simulink model "LinearSolver_System"  (R2021a)
settings: Solver=VariableStepAuto  StartTime=0.0  StopTime=1000  RelTol=1e-3
undefined symbols (not defined in the file or in its folder): AXI4, Lite
libraries: hdlBasic x415, xbsIndex_r4 x1
(part 4 of 4)

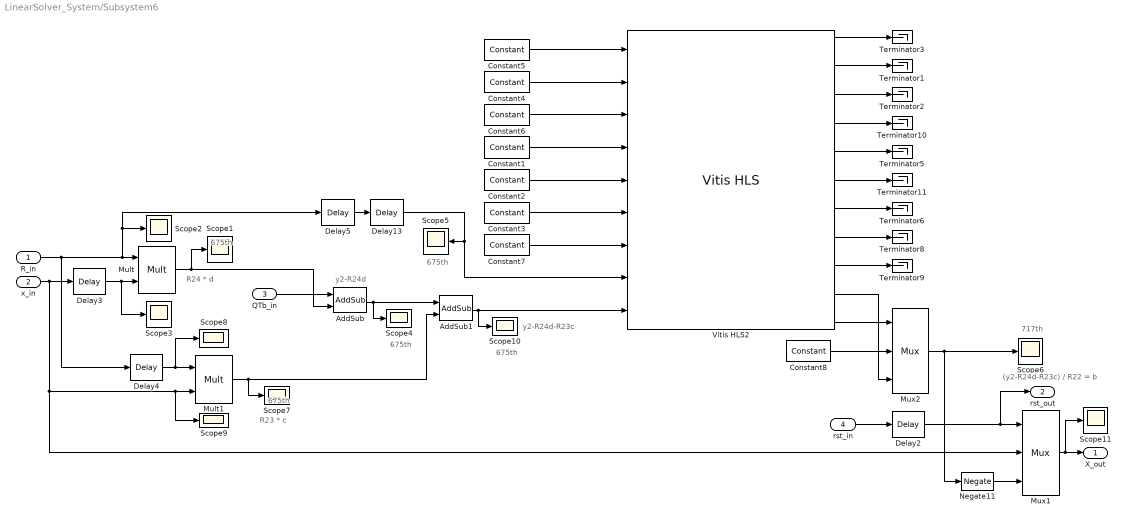
== system LinearSolver_System/Subsystem6 ==
  note: 717th
  note: R24 * d
  note: y2-R24d-R23c
  note: 675th
  note: 675th
  note: (y2-R24d-R23c) / R22 = b
  note: R23 * c
  note: 675th
  note: 675th
  note: 675th
  note: y2-R24d
  R_in : Inport
  x_in : Inport  Port=2
  QTb_in : Inport  Port=3
  rst_in : Inport  Port=4
  AddSub : hdlBasic/AddSub  mode=Subtraction  use_carryin=off  use_carryout=off  en=off  latency=0  precision=User Defined  arith_type="Signed  (2's comp)"  n_bits=16  bin_pt=13  quantization="Round  (unbiased: +/- Inf)"  overflow=Saturate  use_behavioral_HDL=off  hw_selection=Fabric  pipelined=off  XmcBlockStatus=1  maskContainerNames=tabcontainer1  block_type=addsub  block_config=sysgen:Addsub_config
  AddSub1 : hdlBasic/AddSub  mode=Subtraction  use_carryin=off  use_carryout=off  en=off  latency=0  precision=User Defined  arith_type="Signed  (2's comp)"  n_bits=16  bin_pt=13  quantization="Round  (unbiased: +/- Inf)"  overflow=Saturate  use_behavioral_HDL=off  hw_selection=Fabric  pipelined=off  XmcBlockStatus=1  maskContainerNames=tabcontainer1  block_type=addsub  block_config=sysgen:Addsub_config
  Constant{1..3,8} (4 alike) : hdlBasic/Constant  const=0.0  gui_display_data_type=Fixed-point  arith_type=Signed (2's comp)  n_bits=16  bin_pt=13  preci_type=Single  exp_width=8  frac_width=24  explicit_period=off  period=1  XmcBlockStatus=1  maskContainerNames=tabcontainer1  block_type=constant  block_config=sysgen:Constant_config
  Constant4 : hdlBasic/Constant  const=1.0  gui_display_data_type=Boolean  arith_type=Boolean  n_bits=16  bin_pt=14  preci_type=Single  exp_width=8  frac_width=24  explicit_period=off  period=1  XmcBlockStatus=1  maskContainerNames=tabcontainer1  block_type=constant  block_config=sysgen:Constant_config
  Constant5 : hdlBasic/Constant  const=0  gui_display_data_type=Boolean  arith_type=Boolean  n_bits=16  bin_pt=14  preci_type=Single  exp_width=8  frac_width=24  explicit_period=off  period=1  XmcBlockStatus=1  maskContainerNames=tabcontainer1  block_type=constant  block_config=sysgen:Constant_config
  Constant6 : hdlBasic/Constant  const=0  gui_display_data_type=Boolean  arith_type=Boolean  n_bits=16  bin_pt=13  preci_type=Single  exp_width=8  frac_width=24  explicit_period=off  period=1  XmcBlockStatus=1  maskContainerNames=tabcontainer1  block_type=constant  block_config=sysgen:Constant_config
  Constant7 : hdlBasic/Constant  const=0.0  gui_display_data_type=Fixed-point  arith_type=Signed (2's comp)  n_bits=16  bin_pt=0  preci_type=Single  exp_width=8  frac_width=24  explicit_period=off  period=1  XmcBlockStatus=1  maskContainerNames=tabcontainer1  block_type=constant  block_config=sysgen:Constant_config
  Delay{2..5,13} (5 alike) : hdlBasic/Delay  rst=off  en=off  latency=42  reg_retiming=off  XmcBlockStatus=1  maskContainerNames=group1  block_type=delay  block_config=sysgen:Delay_config
  Mult : hdlBasic/Mult  precision=User Defined  arith_type="Signed  (2's comp)"  n_bits=16  bin_pt=13  quantization="Round  (unbiased: +/- Inf)"  overflow=Saturate  en=off  latency=0  use_behavioral_HDL=off  opt=Speed  use_embedded=on  optimum_pipeline=off  pipeline=on  use_rpm=on  placement_style=Triangular  XmcBlockStatus=1  maskContainerNames=group1  block_type=mult  block_config=sysgen:Mult_config
  Mult1 : hdlBasic/Mult  precision=User Defined  arith_type="Signed  (2's comp)"  n_bits=16  bin_pt=13  quantization="Round  (unbiased: +/- Inf)"  overflow=Saturate  en=off  latency=0  use_behavioral_HDL=off  opt=Speed  use_embedded=on  optimum_pipeline=off  pipeline=on  use_rpm=on  placement_style=Triangular  XmcBlockStatus=1  maskContainerNames=group1  block_type=mult  block_config=sysgen:Mult_config
  Mux1 : hdlBasic/Mux  inputs=2  en=off  latency=0  precision=User Defined  arith_type="Signed  (2's comp)"  n_bits=16  bin_pt=13  quantization="Round  (unbiased: +/- Inf)"  overflow=Saturate  XmcBlockStatus=1  maskContainerNames=tabcontainer1  block_type=mux  block_config=sysgen:Mux_config
  Mux2 : hdlBasic/Mux  inputs=2  en=off  latency=0  precision=User Defined  arith_type="Signed  (2's comp)"  n_bits=16  bin_pt=13  quantization="Round  (unbiased: +/- Inf)"  overflow=Saturate  XmcBlockStatus=1  maskContainerNames=tabcontainer1  block_type=mux  block_config=sysgen:Mux_config
  Negate11 : hdlBasic/Negate  precision=User Defined  arith_type="Signed  (2's comp)"  n_bits=16  bin_pt=13  quantization=Truncate  overflow=Wrap  en=off  latency=0  XmcBlockStatus=1  maskContainerNames=tabcontainer1  block_type=negate  block_config=sysgen:Negate_config
  Scope{1..11} (11 alike) : Scope
  Terminator{1..3,5..6,8..11} (9 alike) : Terminator
  Vitis HLS2 : hdlBasic/Vitis HLS  anytable='..\Vitis_HLS\project6_final_hls_mc\solution2_add_back_substitution'  fast_sim=off  display_datatype=off  rate_propagation_method=Simulink system period  model_file_path=''  latency=1  block_type=vitis_hls
      settings: infoedit=This block allows including C,C++ and SystemC source files in System Generator for DSP designs.
  X_out : Outport
  rst_out : Outport  Port=2
  wires:
  Constant4/1 -> Vitis HLS2/2
  Vitis HLS2/4 -> Terminator10/1
  Constant2/1 -> Vitis HLS2/5
  Constant3/1 -> Vitis HLS2/6
  Constant5/1 -> Vitis HLS2/1
  Vitis HLS2/2 -> Terminator1/1
  Vitis HLS2/8 -> Terminator8/1
  Vitis HLS2/9 -> Terminator9/1
  Vitis HLS2/1 -> Terminator3/1
  Constant1/1 -> Vitis HLS2/4
  Constant6/1 -> Vitis HLS2/3
  Constant7/1 -> Vitis HLS2/7
  Vitis HLS2/3 -> Terminator2/1
  Vitis HLS2/5 -> Terminator5/1
  Vitis HLS2/7 -> Terminator6/1
  Vitis HLS2/6 -> Terminator11/1
  QTb_in/1 -> AddSub/1
  R_in/1 -> Delay4/1, Delay5/1, Scope2/1, Mult/1
  Mult/1 -> AddSub/2, Scope1/1
  AddSub/1 -> AddSub1/1, Scope4/1
  Delay13/1 -> Vitis HLS2/8, Scope5/1
  Constant8/1 -> Mux2/2
  Vitis HLS2/10 -> Mux2/3
  Vitis HLS2/11 -> Mux2/1
  rst_in/1 -> Delay2/1
  Delay2/1 -> rst_out/1, Mux1/1
  x_in/1 -> Mux1/2, Scope9/1, Mult1/2, Delay3/1
  Delay3/1 -> Scope3/1, Mult/2
  Mult1/1 -> AddSub1/2, Scope7/1
  Delay4/1 -> Scope8/1, Mult1/1
  AddSub1/1 -> Scope10/1, Vitis HLS2/9
  Delay5/1 -> Delay13/1
  Mux1/1 -> Scope11/1, X_out/1
  Mux2/1 -> Negate11/1, Scope6/1
  Negate11/1 -> Mux1/3

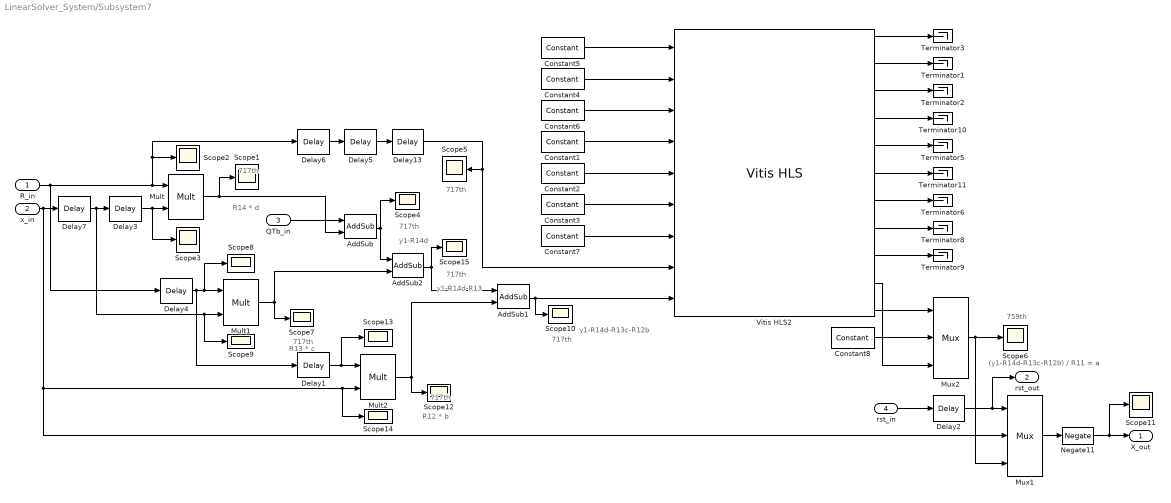
== system LinearSolver_System/Subsystem7 ==
  note: 759th
  note: R14 * d
  note: y1-R14d-R13c-R12b
  note: 717th
  note: 717th
  note: (y1-R14d-R13c-R12b) / R11 = a
  note: R13 * c
  note: 717th
  note: 717th
  note: 717th
  note: y1-R14d
  note: R12 * b
  note: 717th
  note: 717th
  note: y1-R14d-R13
  R_in : Inport
  x_in : Inport  Port=2
  QTb_in : Inport  Port=3
  rst_in : Inport  Port=4
  AddSub : hdlBasic/AddSub  mode=Subtraction  use_carryin=off  use_carryout=off  en=off  latency=0  precision=User Defined  arith_type="Signed  (2's comp)"  n_bits=16  bin_pt=13  quantization="Round  (unbiased: +/- Inf)"  overflow=Saturate  use_behavioral_HDL=off  hw_selection=Fabric  pipelined=off  XmcBlockStatus=1  maskContainerNames=tabcontainer1  block_type=addsub  block_config=sysgen:Addsub_config
  AddSub1 : hdlBasic/AddSub  mode=Subtraction  use_carryin=off  use_carryout=off  en=off  latency=0  precision=User Defined  arith_type="Signed  (2's comp)"  n_bits=16  bin_pt=13  quantization="Round  (unbiased: +/- Inf)"  overflow=Saturate  use_behavioral_HDL=off  hw_selection=Fabric  pipelined=off  XmcBlockStatus=1  maskContainerNames=tabcontainer1  block_type=addsub  block_config=sysgen:Addsub_config
  AddSub2 : hdlBasic/AddSub  mode=Subtraction  use_carryin=off  use_carryout=off  en=off  latency=0  precision=User Defined  arith_type="Signed  (2's comp)"  n_bits=16  bin_pt=13  quantization="Round  (unbiased: +/- Inf)"  overflow=Saturate  use_behavioral_HDL=off  hw_selection=Fabric  pipelined=off  XmcBlockStatus=1  maskContainerNames=tabcontainer1  block_type=addsub  block_config=sysgen:Addsub_config
  Constant{1..3,8} (4 alike) : hdlBasic/Constant  const=0.0  gui_display_data_type=Fixed-point  arith_type=Signed (2's comp)  n_bits=16  bin_pt=13  preci_type=Single  exp_width=8  frac_width=24  explicit_period=off  period=1  XmcBlockStatus=1  maskContainerNames=tabcontainer1  block_type=constant  block_config=sysgen:Constant_config
  Constant4 : hdlBasic/Constant  const=1.0  gui_display_data_type=Boolean  arith_type=Boolean  n_bits=16  bin_pt=14  preci_type=Single  exp_width=8  frac_width=24  explicit_period=off  period=1  XmcBlockStatus=1  maskContainerNames=tabcontainer1  block_type=constant  block_config=sysgen:Constant_config
  Constant5 : hdlBasic/Constant  const=0  gui_display_data_type=Boolean  arith_type=Boolean  n_bits=16  bin_pt=14  preci_type=Single  exp_width=8  frac_width=24  explicit_period=off  period=1  XmcBlockStatus=1  maskContainerNames=tabcontainer1  block_type=constant  block_config=sysgen:Constant_config
  Constant6 : hdlBasic/Constant  const=0  gui_display_data_type=Boolean  arith_type=Boolean  n_bits=16  bin_pt=13  preci_type=Single  exp_width=8  frac_width=24  explicit_period=off  period=1  XmcBlockStatus=1  maskContainerNames=tabcontainer1  block_type=constant  block_config=sysgen:Constant_config
  Constant7 : hdlBasic/Constant  const=0.0  gui_display_data_type=Fixed-point  arith_type=Signed (2's comp)  n_bits=16  bin_pt=0  preci_type=Single  exp_width=8  frac_width=24  explicit_period=off  period=1  XmcBlockStatus=1  maskContainerNames=tabcontainer1  block_type=constant  block_config=sysgen:Constant_config
  Delay{1..7,13} (8 alike) : hdlBasic/Delay  rst=off  en=off  latency=42  reg_retiming=off  XmcBlockStatus=1  maskContainerNames=group1  block_type=delay  block_config=sysgen:Delay_config
  Mult : hdlBasic/Mult  precision=User Defined  arith_type="Signed  (2's comp)"  n_bits=16  bin_pt=13  quantization="Round  (unbiased: +/- Inf)"  overflow=Saturate  en=off  latency=0  use_behavioral_HDL=off  opt=Speed  use_embedded=on  optimum_pipeline=off  pipeline=on  use_rpm=on  placement_style=Triangular  XmcBlockStatus=1  maskContainerNames=group1  block_type=mult  block_config=sysgen:Mult_config
  Mult1 : hdlBasic/Mult  precision=User Defined  arith_type="Signed  (2's comp)"  n_bits=16  bin_pt=13  quantization="Round  (unbiased: +/- Inf)"  overflow=Saturate  en=off  latency=0  use_behavioral_HDL=off  opt=Speed  use_embedded=on  optimum_pipeline=off  pipeline=on  use_rpm=on  placement_style=Triangular  XmcBlockStatus=1  maskContainerNames=group1  block_type=mult  block_config=sysgen:Mult_config
  Mult2 : hdlBasic/Mult  precision=User Defined  arith_type="Signed  (2's comp)"  n_bits=16  bin_pt=13  quantization="Round  (unbiased: +/- Inf)"  overflow=Saturate  en=off  latency=0  use_behavioral_HDL=off  opt=Speed  use_embedded=on  optimum_pipeline=off  pipeline=on  use_rpm=on  placement_style=Triangular  XmcBlockStatus=1  maskContainerNames=group1  block_type=mult  block_config=sysgen:Mult_config
  Mux1 : hdlBasic/Mux  inputs=2  en=off  latency=0  precision=Full  arith_type="Signed  (2's comp)"  n_bits=16  bin_pt=13  quantization="Round  (unbiased: +/- Inf)"  overflow=Saturate  XmcBlockStatus=1  maskContainerNames=tabcontainer1  block_type=mux  block_config=sysgen:Mux_config
  Mux2 : hdlBasic/Mux  inputs=2  en=off  latency=0  precision=User Defined  arith_type="Signed  (2's comp)"  n_bits=16  bin_pt=13  quantization="Round  (unbiased: +/- Inf)"  overflow=Saturate  XmcBlockStatus=1  maskContainerNames=tabcontainer1  block_type=mux  block_config=sysgen:Mux_config
  Negate11 : hdlBasic/Negate  precision=User Defined  arith_type="Signed  (2's comp)"  n_bits=16  bin_pt=13  quantization=Truncate  overflow=Wrap  en=off  latency=0  XmcBlockStatus=1  maskContainerNames=tabcontainer1  block_type=negate  block_config=sysgen:Negate_config
  Scope{1..15} (15 alike) : Scope
  Terminator{1..3,5..6,8..11} (9 alike) : Terminator
  Vitis HLS2 : hdlBasic/Vitis HLS  anytable='..\Vitis_HLS\project6_final_hls_mc\solution2_add_back_substitution'  fast_sim=off  display_datatype=off  rate_propagation_method=Simulink system period  model_file_path=''  latency=1  block_type=vitis_hls
      settings: infoedit=This block allows including C,C++ and SystemC source files in System Generator for DSP designs.
  X_out : Outport
  rst_out : Outport  Port=2
  wires:
  Constant4/1 -> Vitis HLS2/2
  Vitis HLS2/4 -> Terminator10/1
  Constant2/1 -> Vitis HLS2/5
  Constant3/1 -> Vitis HLS2/6
  Constant5/1 -> Vitis HLS2/1
  Vitis HLS2/2 -> Terminator1/1
  Vitis HLS2/8 -> Terminator8/1
  Vitis HLS2/9 -> Terminator9/1
  Vitis HLS2/1 -> Terminator3/1
  Constant1/1 -> Vitis HLS2/4
  Constant6/1 -> Vitis HLS2/3
  Constant7/1 -> Vitis HLS2/7
  Vitis HLS2/3 -> Terminator2/1
  Vitis HLS2/5 -> Terminator5/1
  Vitis HLS2/7 -> Terminator6/1
  Vitis HLS2/6 -> Terminator11/1
  QTb_in/1 -> AddSub/1
  R_in/1 -> Delay6/1, Scope2/1, Mult/1, Delay4/1
  Mult/1 -> AddSub/2, Scope1/1
  AddSub/1 -> AddSub2/1, Scope4/1
  Delay13/1 -> Vitis HLS2/8, Scope5/1
  Constant8/1 -> Mux2/2
  Vitis HLS2/10 -> Mux2/3
  Vitis HLS2/11 -> Mux2/1
  rst_in/1 -> Delay2/1
  Delay2/1 -> rst_out/1, Mux1/1
  x_in/1 -> Scope14/1, Mult2/2, Mux1/2, Delay7/1
  Delay3/1 -> Scope3/1, Mult/2
  Mult1/1 -> AddSub2/2, Scope7/1
  Delay4/1 -> Delay1/1, Scope8/1, Mult1/1
  AddSub1/1 -> Scope10/1, Vitis HLS2/9
  Delay5/1 -> Delay13/1
  Mult2/1 -> AddSub1/2, Scope12/1
  Delay1/1 -> Scope13/1, Mult2/1
  AddSub2/1 -> AddSub1/1, Scope15/1
  Delay6/1 -> Delay5/1
  Delay7/1 -> Scope9/1, Mult1/2, Delay3/1
  Mux2/1 -> Mux1/3, Scope6/1
  Mux1/1 -> Negate11/1
  Negate11/1 -> Scope11/1, X_out/1
